simulink model "Mtest6"  (R2021b)
settings: Solver=FixedStepDiscrete  StartTime=0.0  StopTime=t_sim  FixedStep=0.01  RelTol=1e-3  EnableMultiTasking=on
model workspace (MAT data in the model file):
  SL_ROS_VariableLengthArrays_MaxSizes.CommonInfo.ArrayTruncateAction = 'EmitWarning'
  SL_ROS_VariableLengthArrays_MaxSizes.MsgTypeMap = containers.Map
  SL_ROS_VariableLengthArrays_MaxSizes.MsgTypeMap.serialization.keys = {'sensor_msgs/LaserScan'}
  SL_ROS_VariableLengthArrays_MaxSizes.MsgTypeMap.serialization.values{1}(1).PropertyName = 'Intensities'
  SL_ROS_VariableLengthArrays_MaxSizes.MsgTypeMap.serialization.values{1}(1).DataType = 'single'
  SL_ROS_VariableLengthArrays_MaxSizes.MsgTypeMap.serialization.values{1}(1).MaxLength = 360
  SL_ROS_VariableLengthArrays_MaxSizes.MsgTypeMap.serialization.values{1}(2).PropertyName = 'Ranges'
  SL_ROS_VariableLengthArrays_MaxSizes.MsgTypeMap.serialization.values{1}(2).DataType = 'single'
  SL_ROS_VariableLengthArrays_MaxSizes.MsgTypeMap.serialization.values{1}(2).MaxLength = 360
  SL_ROS_VariableLengthArrays_MaxSizes.MsgTypeMap.serialization.uniformity = 0
  SL_ROS_VariableLengthArrays_MaxSizes.MsgTypeMap.serialization.keyType = 'char'
  SL_ROS_VariableLengthArrays_MaxSizes.MsgTypeMap.serialization.valueType = 'any'
  rampa = 1
values from neighbouring files (symbols this model uses):
  x = x-0.1    [movimiento.m]
  y = y-0.1    [movimiento.m]
undefined symbols (not defined in the file or in its folder): a, Angular, Linear, rx1, rx2, rx3, ry1, ry2, ry3
libraries: robotlib x14, robotcorelib x3, robotalgslib x3, instrumentlib x1
settings Model: PacingRate=0.450000  Creator=The MathWorks, Inc.  LastModifiedBy=Cinthy
settings SolverCC: ConcurrentTasks=on  AlgebraicLoopSolver=TrustRegion  AutoInsertRateTranBlk=on
settings DataIOCC: LimitDataPoints=on  SaveFormat=StructureWithTime  ReturnWorkspaceOutputs=off
settings OptimizationCC: BlockReduction=off  EnhancedBackFolding=on  PassReuseOutputArgsAs=Individual arguments  ZeroExternalMemoryAtStartup=off  ZeroInternalMemoryAtStartup=off  MaxStackSize=64  OptimizeBlockOrder=speed  DifferentSizesBufferReuse=on  OptimizationCustomize=off  EfficientTunableParamExpr=on
settings DebuggingCC: SolverPrmCheckMsg=warning  ParameterTunabilityLossMsg=error  SFUnexpectedBacktrackingDiag=warning  SFNoUnconditionalDefaultTransitionDiag=warning  SFExecutionAtInitializationDiag=none  SFMachineParentedDataDiag=warning  ArithmeticOperatorsInVariantConditions=warning
settings HardwareCC: ProdBitPerPointer=32  ProdBitPerSizeT=32  ProdBitPerPtrDiffT=32  ProdLargestAtomicFloat=None  ProdIntDivRoundTo=Undefined  ProdEndianess=Unspecified  ProdWordSize=32  ProdHWDeviceType=Generic->Unspecified (assume 32-bit Generic)  TargetHWDeviceType=Generic->Unspecified (assume 32-bit Generic)
settings ModelReferenceCC: ModelReferenceNumInstancesAllowed=Single  PropagateSignalLabelsOutOfModel=off
settings SFSimCC: SimUseLocalCustomCode=off  MATLABDynamicMemAlloc=off  CustomCodeUndefinedFunction=UseInterfaceOnly  SimTargetLang=C++
settings RTWCC: Description=Embedded Coder  SystemTargetFile=ert.tlc  HardwareBoard=Robot Operating System (ROS)  TLCOptions="-aInlineSetEventsForThisBaseRateFcn=TLC_FALSE -aSuppressMultiTaskScheduler=TLC_FALSE  -aRateBasedStepFcn=0"  TemplateMakefile=ert_default_tmf  RTWUseLocalCustomCode=off  Toolchain=Catkin  TargetLang=C++
settings CodeAppCC: ForceParamTrailComments=on  IgnoreCustomStorageClasses=off  OperatorAnnotations=on  SimulinkDataObjDesc=on  SFDataObjDesc=on  InsertBlockDesc=on
settings ConfigComp: CovMetricSettings=dw  CovSaveCumulativeToWorkspaceVar=on  CovSaveSingleToWorkspaceVar=on  CovExternalEMLEnable=off  CovSFcnEnable=off

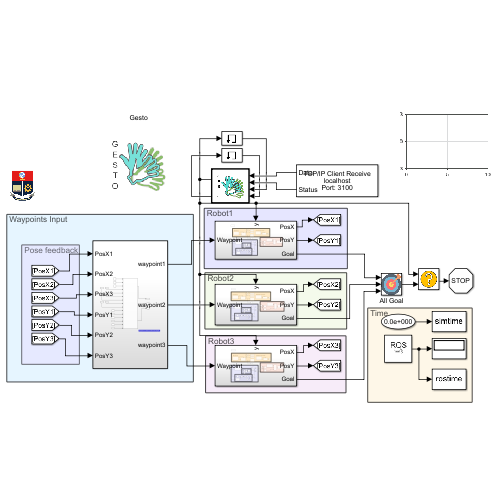
[thumbnail: Simulink's stored preview of the top-level diagram]
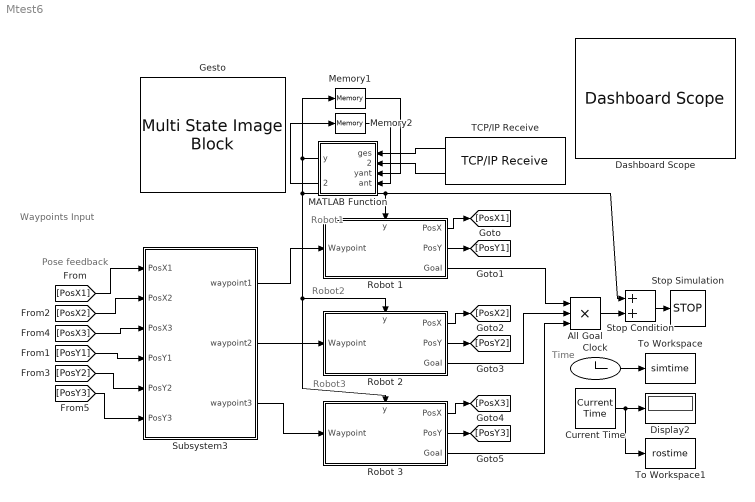
== system Mtest6 ==
  note: Time
  note: Pose feedback
  note: Robot3
  note: Robot2
  note: Robot1
  note: Waypoints Input
  All Goal : Product  Inputs=3  OutDataTypeStr=double
      mask Display: image('$imagefile'); % Use "Edit Image" on toolstrip to change.
  Clock : Clock
  Current Time : robotlib/Current Time  OutputFormat=double  SampleTime=-1  ModelName=Mtest6
      settings: SourceProductBaseCode=RR
  Dashboard Scope : DashboardScope  NormalizeYAxis=on
  Display2 : Display
  Gesto : MultiStateImageBlock  LabelPosition=Hide
  MATLAB Function : MATLAB Function  TreatAsAtomicUnit=on
  Memory1 : Memory
  Memory2 : Memory
  Robot 1 : Subsystem
      settings: PortSchema="{\"entries\":[{\"content\":{\"sides\":[{\"content\":{\"connectorIds\":[\"In1\"]},\"type\":\"ConnectorPlacement.EquallySpacedRectSide\",\"uuid\":\"ae525184-150a-424a-8495-0e96f94f0405\"},{\"content\":{\"connectorIds\":[\"Out1\",\"Out2\",\"Out3\"],\"side\":\"RIGHT\"},\"type\":\"ConnectorPlacement.EquallySpacedRectSide\",\"uuid\":\"56be0739-f54c-4565-abf9-53a283bf784a\"},{\"content\":{\"connectorIds\":[\"In2\"],\"side\":\"TOP\"},\"type\":\"ConnectorPlacement.EquallySpacedRectSide\",\"uuid\":\"def6bcfa-390a-4ec0-9486-bcadb35013bb\"}]},\"type\":\"ConnectorPlacement.EquallySpacedConnector\",\"uuid\":\"b414c082-bc88-4d09-823a-fc3316a4064c\"}],\"packageUris\":[\"http://schema.mathworks.com/mf0/Connector/R2020b\"],\"version\":\"1.0\"}"
  Robot 2 : Subsystem
      settings: PortSchema="{\"entries\":[{\"content\":{\"sides\":[{\"content\":{\"connectorIds\":[\"In1\"]},\"type\":\"ConnectorPlacement.EquallySpacedRectSide\",\"uuid\":\"ae525184-150a-424a-8495-0e96f94f0405\"},{\"content\":{\"connectorIds\":[\"Out1\",\"Out2\",\"Out3\"],\"side\":\"RIGHT\"},\"type\":\"ConnectorPlacement.EquallySpacedRectSide\",\"uuid\":\"56be0739-f54c-4565-abf9-53a283bf784a\"},{\"content\":{\"connectorIds\":[\"In2\"],\"side\":\"TOP\"},\"type\":\"ConnectorPlacement.EquallySpacedRectSide\",\"uuid\":\"def6bcfa-390a-4ec0-9486-bcadb35013bb\"}]},\"type\":\"ConnectorPlacement.EquallySpacedConnector\",\"uuid\":\"b414c082-bc88-4d09-823a-fc3316a4064c\"}],\"packageUris\":[\"http://schema.mathworks.com/mf0/Connector/R2020b\"],\"version\":\"1.0\"}"
  Robot 3 : Subsystem
      settings: PortSchema="{\"entries\":[{\"content\":{\"sides\":[{\"content\":{\"connectorIds\":[\"In1\"]},\"type\":\"ConnectorPlacement.EquallySpacedRectSide\",\"uuid\":\"ae525184-150a-424a-8495-0e96f94f0405\"},{\"content\":{\"connectorIds\":[\"Out1\",\"Out2\",\"Out3\"],\"side\":\"RIGHT\"},\"type\":\"ConnectorPlacement.EquallySpacedRectSide\",\"uuid\":\"56be0739-f54c-4565-abf9-53a283bf784a\"},{\"content\":{\"connectorIds\":[\"In2\"],\"side\":\"TOP\"},\"type\":\"ConnectorPlacement.EquallySpacedRectSide\",\"uuid\":\"def6bcfa-390a-4ec0-9486-bcadb35013bb\"}]},\"type\":\"ConnectorPlacement.EquallySpacedConnector\",\"uuid\":\"b414c082-bc88-4d09-823a-fc3316a4064c\"}],\"packageUris\":[\"http://schema.mathworks.com/mf0/Connector/R2020b\"],\"version\":\"1.0\"}"
  Stop Condition : Sum
      mask Display: image('$imagefile'); % Use "Edit Image" on toolstrip to change.
  Stop Simulation : Stop
  Subsystem3 : Subsystem
  TCP/IP Receive : instrumentlib/TCP//IP Receive  Host=localhost  Port=3100  DataSize=[ 1, 1 ]  DataType=uint8  ASCIIFormatting=%f  Terminator=LF  CustomTerminator=10  ByteOrder=big-endian  EnableBlockingMode=off  Timeout=10  SampleTime=0.1  SimulateUsing=Interpreted execution
  To Workspace : ToWorkspace  VariableName=simtime  SampleTime=-1
  To Workspace1 : ToWorkspace  VariableName=rostime  SampleTime=-1
  wires:
  Robot 1/1(PosX) -> [PosX1]
  Robot 1/2(PosY) -> [PosY1]
  Robot 2/1(PosX) -> [PosX2]
  Robot 2/2(PosY) -> [PosY2]
  Robot 3/1(PosX) -> [PosX3]
  Robot 3/2(PosY) -> [PosY3]
  Subsystem3/1(waypoint1) -> Robot 1/1(Waypoint)
  Subsystem3/2(waypoint2) -> Robot 2/1(Waypoint)
  Subsystem3/3(waypoint3) -> Robot 3/1(Waypoint)
  Robot 1/3(Goal) -> All Goal/1
  Robot 2/3(Goal) -> All Goal/2
  Robot 3/3(Goal) -> All Goal/3
  Clock/1 -> To Workspace/1
  [PosX1] -> Subsystem3/1(PosX1)
  [PosX2] -> Subsystem3/2(PosX2)
  [PosX3] -> Subsystem3/3(PosX3)
  [PosY1] -> Subsystem3/4(PosY1)
  [PosY2] -> Subsystem3/5(PosY2)
  [PosY3] -> Subsystem3/6(PosY3)
  Current Time/1 -> To Workspace1/1, Display2/1
  TCP/IP Receive/1 -> MATLAB Function/1(ges)
  MATLAB Function/1(y) -> Memory1/1, Robot 1/2(y), Stop Condition/1, Robot 2/2(y), Robot 3/2(y)
  All Goal/1 -> Stop Condition/2
  Stop Condition/1 -> Stop Simulation/1
  TCP/IP Receive/2 -> MATLAB Function/2(newData)
  MATLAB Function/2(gesto) -> Memory2/1
  Memory1/1 -> MATLAB Function/3(yant)
  Memory2/1 -> MATLAB Function/4(ant)

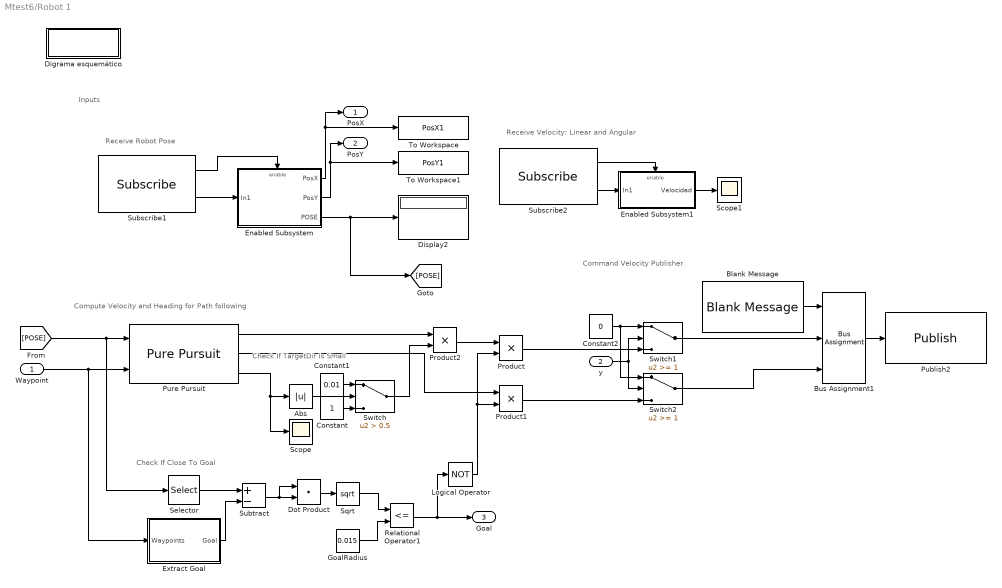
== system Mtest6/Robot 1 ==
  note: Check If TargetDir Is Small
  note: Compute Velocity and Heading for Path following
  note: Inputs
  note: Receive Robot Pose
  note: Check If Close To Goal
  note: Command Velocity Publisher
  note: Receive Velocity: Linear and Angular
  Waypoint : Inport
  y : Inport  Port=2
  " Extract Goal" : MATLAB Function  TreatAsAtomicUnit=on
  Abs : Abs
  Blank Message : robotlib/Blank Message  messageClass=Message  entityType=geometry_msgs/Twist  messageType=geometry_msgs/Twist  SampleTime=inf  legacyBusStruct=off
  Bus Assignment1 : BusAssignment  DialogController=Simulink.DDGSource_BusAssignment  AssignedSignals=Linear.X,Angular.Z
  Constant : Constant
  Constant1 : Constant  Value=0.01
  Constant2 : Constant  Value=0
  Digrama esquemático : Subsystem
  Display2 : Display
  Dot Product : DotProduct  InputSameDT=on  OutDataTypeStr=Inherit: Inherit via internal rule
  Enabled Subsystem : Subsystem
  Enabled Subsystem1 : Subsystem
  GoalRadius : Constant  Value=0.015
  Logical Operator : Logic  Operator=NOT  AllPortsSameDT=off  OutDataTypeStr=boolean
  Product : Product
  Product1 : Product
  Product2 : Product
  Publish2 : robotlib/Publish  topicSource=Select from ROS network  topic=/robot1/cmd_vel  messageType=geometry_msgs/Twist  legacyBusStruct=off  messageQueueLength=105
  Pure Pursuit : robotalgslib/Pure Pursuit  DesiredLinearVelocity=0.22  MaxAngularVelocity=2.84  LookaheadDistance=1.0  TargetDirPort=on  SimulateUsing=Code generation
  Relational Operator1 : RelationalOperator  Operator=<=  OutDataTypeStr=boolean  RndMeth=Simplest
  Scope : Scope
  Scope1 : Scope
  Selector : Selector  InputPortWidth=3  IndexOptions=Index vector (dialog)  Indices=[1 2]  OutputSizes=1
  Sqrt : Sqrt  SaturateOnIntegerOverflow=on
  Subscribe1 : robotlib/Subscribe  topicSource=Select from ROS network  topic=/robot1/odom  messageType=nav_msgs/Odometry  SampleTime=-1  legacyBusStruct=off  messageQueueLength=51
  Subscribe2 : robotlib/Subscribe  topicSource=Select from ROS network  topic=/robot1/cmd_vel  messageType=geometry_msgs/Twist  SampleTime=-1  legacyBusStruct=off  messageQueueLength=51
  Subtract : Sum  Inputs=+-
  Switch : Switch  Criteria=u2 > Threshold  Threshold=0.5
  Switch1 : Switch  Threshold=1
  Switch2 : Switch  Threshold=1
  To Workspace : ToWorkspace  VariableName=PosX1  SampleTime=-1
  To Workspace1 : ToWorkspace  VariableName=PosY1  SampleTime=-1
  PosX : Outport
  PosY : Outport  Port=2
  Goal : Outport  Port=3
  wires:
  GoalRadius/1 -> Relational Operator1/2
  Blank Message/1 -> Bus Assignment1/1
  Enabled Subsystem/3(POSE) -> [POSE], Display2/1
  Subtract/1 -> Dot Product/1, Dot Product/2
  Enabled Subsystem/2(PosY) -> PosY/1, To Workspace1/1
  Subscribe1/2 -> Enabled Subsystem/1(In1)
  Pure Pursuit/2 -> Product1/1
  Subscribe1/1 -> Enabled Subsystem/Enable
  Enabled Subsystem/1(PosX) -> PosX/1, To Workspace/1
  Relational Operator1/1 -> Logical Operator/1, Goal/1
  Bus Assignment1/1 -> Publish2/1
  [POSE] -> Selector/1, Pure Pursuit/1
  Dot Product/1 -> Sqrt/1
  " Extract Goal"/1(Goal) -> Subtract/2
  Selector/1 -> Subtract/1
  Sqrt/1 -> Relational Operator1/1
  Logical Operator/1 -> Product/2, Product1/2
  Waypoint/1 -> " Extract Goal"/1(Waypoints), Pure Pursuit/2
  Pure Pursuit/3 -> Scope/1, Abs/1
  Constant/1 -> Switch/3
  Constant1/1 -> Switch/1
  Switch/1 -> Product2/2
  Product2/1 -> Product/1
  Abs/1 -> Switch/2
  Pure Pursuit/1 -> Product2/1
  y/1 -> Switch1/2, Switch2/2
  Constant2/1 -> Switch2/1, Switch1/1
  Product/1 -> Switch1/3
  Product1/1 -> Switch2/3
  Switch1/1 -> Bus Assignment1/2
  Switch2/1 -> Bus Assignment1/3
  Subscribe2/2 -> Enabled Subsystem1/1(In1)
  Subscribe2/1 -> Enabled Subsystem1/Enable
  Enabled Subsystem1/1(Velocidad) -> Scope1/1

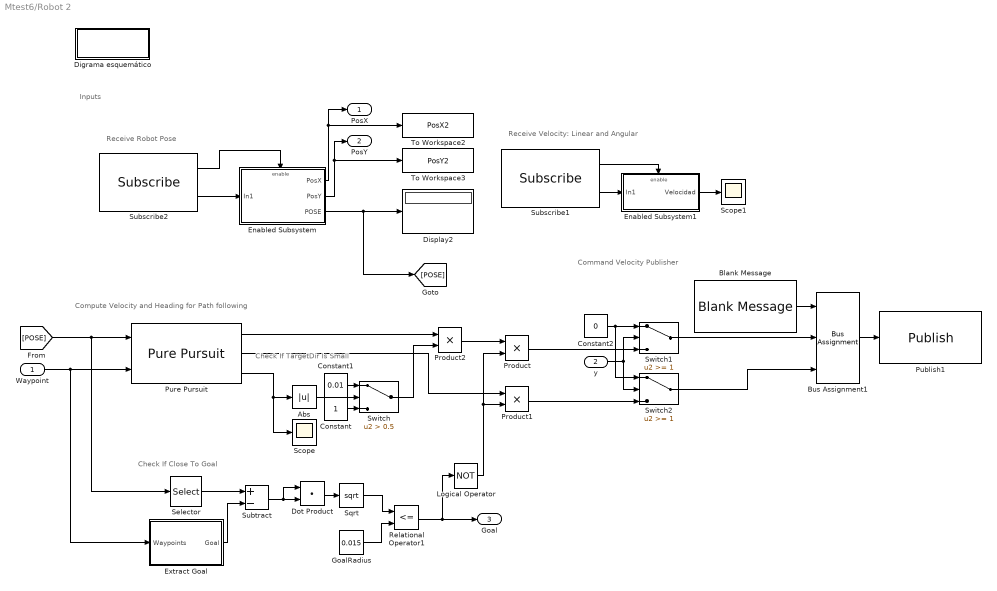
== system Mtest6/Robot 2 ==
  note: Check If TargetDir Is Small
  note: Compute Velocity and Heading for Path following
  note: Inputs
  note: Receive Robot Pose
  note: Check If Close To Goal
  note: Command Velocity Publisher
  note: Receive Velocity: Linear and Angular
  Waypoint : Inport
  y : Inport  Port=2
  " Extract Goal" : MATLAB Function  TreatAsAtomicUnit=on
  Abs : Abs
  Blank Message : robotlib/Blank Message  messageClass=Message  entityType=geometry_msgs/Twist  messageType=geometry_msgs/Twist  SampleTime=inf  legacyBusStruct=off
  Bus Assignment1 : BusAssignment  DialogController=Simulink.DDGSource_BusAssignment  AssignedSignals=Linear.X,Angular.Z
  Constant : Constant
  Constant1 : Constant  Value=0.01
  Constant2 : Constant  Value=0
  Digrama esquemático : Subsystem
  Display2 : Display
  Dot Product : DotProduct  InputSameDT=on  OutDataTypeStr=Inherit: Inherit via internal rule
  Enabled Subsystem : Subsystem
  Enabled Subsystem1 : Subsystem
  GoalRadius : Constant  Value=0.015
  Logical Operator : Logic  Operator=NOT  AllPortsSameDT=off  OutDataTypeStr=boolean
  Product : Product
  Product1 : Product
  Product2 : Product
  Publish1 : robotlib/Publish  topicSource=Select from ROS network  topic=/robot2/cmd_vel  messageType=geometry_msgs/Twist  legacyBusStruct=off  messageQueueLength=105
  Pure Pursuit : robotalgslib/Pure Pursuit  DesiredLinearVelocity=0.22  MaxAngularVelocity=2.84  LookaheadDistance=1.0  TargetDirPort=on  SimulateUsing=Code generation
  Relational Operator1 : RelationalOperator  Operator=<=  OutDataTypeStr=boolean  RndMeth=Simplest
  Scope : Scope
  Scope1 : Scope
  Selector : Selector  InputPortWidth=3  IndexOptions=Index vector (dialog)  Indices=[1 2]  OutputSizes=1
  Sqrt : Sqrt  SaturateOnIntegerOverflow=on
  Subscribe1 : robotlib/Subscribe  topicSource=Select from ROS network  topic=/robot2/cmd_vel  messageType=geometry_msgs/Twist  SampleTime=-1  legacyBusStruct=off  messageQueueLength=51
  Subscribe2 : robotlib/Subscribe  topicSource=Select from ROS network  topic=/robot2/odom  messageType=nav_msgs/Odometry  SampleTime=-1  legacyBusStruct=off  messageQueueLength=51
  Subtract : Sum  Inputs=+-
  Switch : Switch  Criteria=u2 > Threshold  Threshold=0.5
  Switch1 : Switch  Threshold=1
  Switch2 : Switch  Threshold=1
  To Workspace2 : ToWorkspace  VariableName=PosX2  SampleTime=-1
  To Workspace3 : ToWorkspace  VariableName=PosY2  SampleTime=-1
  PosX : Outport
  PosY : Outport  Port=2
  Goal : Outport  Port=3
  wires:
  GoalRadius/1 -> Relational Operator1/2
  Blank Message/1 -> Bus Assignment1/1
  Enabled Subsystem/3(POSE) -> [POSE], Display2/1
  Subtract/1 -> Dot Product/1, Dot Product/2
  Enabled Subsystem/2(PosY) -> To Workspace3/1, PosY/1
  Subscribe2/2 -> Enabled Subsystem/1(In1)
  Pure Pursuit/2 -> Product1/1
  Subscribe2/1 -> Enabled Subsystem/Enable
  Enabled Subsystem/1(PosX) -> To Workspace2/1, PosX/1
  Relational Operator1/1 -> Logical Operator/1, Goal/1
  Bus Assignment1/1 -> Publish1/1
  [POSE] -> Selector/1, Pure Pursuit/1
  Dot Product/1 -> Sqrt/1
  " Extract Goal"/1(Goal) -> Subtract/2
  Selector/1 -> Subtract/1
  Sqrt/1 -> Relational Operator1/1
  Logical Operator/1 -> Product/2, Product1/2
  Waypoint/1 -> " Extract Goal"/1(Waypoints), Pure Pursuit/2
  Pure Pursuit/3 -> Scope/1, Abs/1
  Constant/1 -> Switch/3
  Constant1/1 -> Switch/1
  Switch/1 -> Product2/2
  Product2/1 -> Product/1
  Abs/1 -> Switch/2
  Pure Pursuit/1 -> Product2/1
  Product1/1 -> Switch2/3
  y/1 -> Switch1/2, Switch2/2
  Constant2/1 -> Switch2/1, Switch1/1
  Product/1 -> Switch1/3
  Switch1/1 -> Bus Assignment1/2
  Switch2/1 -> Bus Assignment1/3
  Subscribe1/1 -> Enabled Subsystem1/Enable
  Subscribe1/2 -> Enabled Subsystem1/1(In1)
  Enabled Subsystem1/1(Velocidad) -> Scope1/1

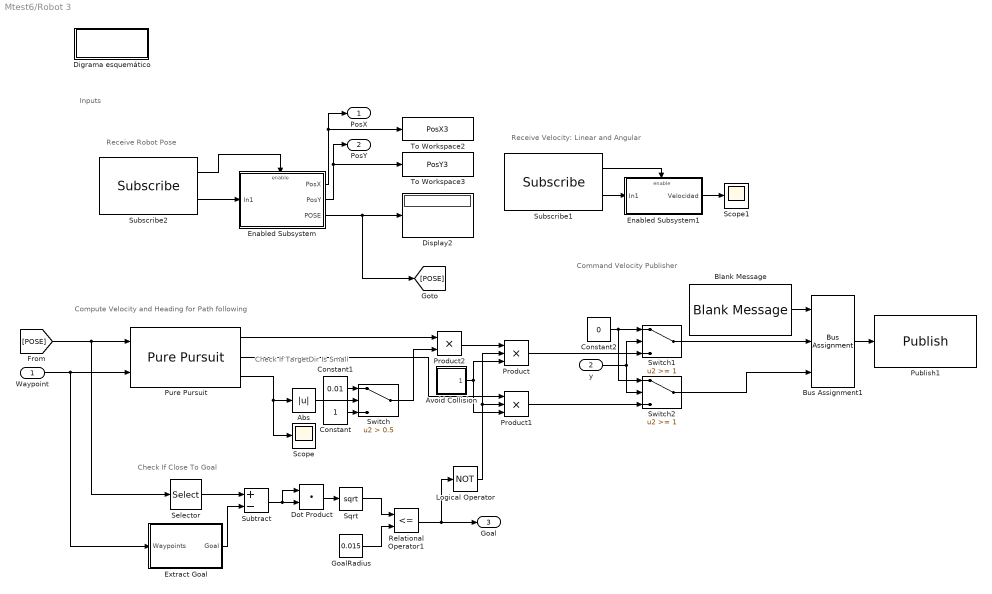
== system Mtest6/Robot 3 ==
  note: Check If TargetDir Is Small
  note: Compute Velocity and Heading for Path following
  note: Inputs
  note: Receive Robot Pose
  note: Check If Close To Goal
  note: Command Velocity Publisher
  note: Receive Velocity: Linear and Angular
  Waypoint : Inport
  y : Inport  Port=2
  " Extract Goal" : MATLAB Function  TreatAsAtomicUnit=on
  Abs : Abs
  Avoid Collision : Subsystem
  Blank Message : robotlib/Blank Message  messageClass=Message  entityType=geometry_msgs/Twist  messageType=geometry_msgs/Twist  SampleTime=inf  legacyBusStruct=off
  Bus Assignment1 : BusAssignment  DialogController=Simulink.DDGSource_BusAssignment  AssignedSignals=Linear.X,Angular.Z
  Constant : Constant
  Constant1 : Constant  Value=0.01
  Constant2 : Constant  Value=0
  Digrama esquemático : Subsystem
  Display2 : Display
  Dot Product : DotProduct  InputSameDT=on  OutDataTypeStr=Inherit: Inherit via internal rule
  Enabled Subsystem : Subsystem
  Enabled Subsystem1 : Subsystem
  GoalRadius : Constant  Value=0.015
  Logical Operator : Logic  Operator=NOT  AllPortsSameDT=off  OutDataTypeStr=boolean
  Product : Product  Inputs=3
  Product1 : Product  Inputs=3
  Product2 : Product
  Publish1 : robotlib/Publish  topicSource=Select from ROS network  topic=/robot3/cmd_vel  messageType=geometry_msgs/Twist  legacyBusStruct=off  messageQueueLength=105
  Pure Pursuit : robotalgslib/Pure Pursuit  DesiredLinearVelocity=0.22  MaxAngularVelocity=2.84  LookaheadDistance=1.0  TargetDirPort=on  SimulateUsing=Code generation
  Relational Operator1 : RelationalOperator  Operator=<=  OutDataTypeStr=boolean  RndMeth=Simplest
  Scope : Scope
  Scope1 : Scope
  Selector : Selector  InputPortWidth=3  IndexOptions=Index vector (dialog)  Indices=[1 2]  OutputSizes=1
  Sqrt : Sqrt  SaturateOnIntegerOverflow=on
  Subscribe1 : robotlib/Subscribe  topicSource=Select from ROS network  topic=/robot3/cmd_vel  messageType=geometry_msgs/Twist  SampleTime=-1  legacyBusStruct=off  messageQueueLength=51
  Subscribe2 : robotlib/Subscribe  topicSource=Select from ROS network  topic=/robot3/odom  messageType=nav_msgs/Odometry  SampleTime=-1  legacyBusStruct=off  messageQueueLength=51
  Subtract : Sum  Inputs=+-
  Switch : Switch  Criteria=u2 > Threshold  Threshold=0.5
  Switch1 : Switch  Threshold=1
  Switch2 : Switch  Threshold=1
  To Workspace2 : ToWorkspace  VariableName=PosX3  SampleTime=-1
  To Workspace3 : ToWorkspace  VariableName=PosY3  SampleTime=-1
  PosX : Outport
  PosY : Outport  Port=2
  Goal : Outport  Port=3
  wires:
  GoalRadius/1 -> Relational Operator1/2
  Blank Message/1 -> Bus Assignment1/1
  Enabled Subsystem/3(POSE) -> [POSE], Display2/1
  Subtract/1 -> Dot Product/1, Dot Product/2
  Enabled Subsystem/2(PosY) -> To Workspace3/1, PosY/1
  Subscribe2/2 -> Enabled Subsystem/1(In1)
  Pure Pursuit/2 -> Product1/1
  Subscribe2/1 -> Enabled Subsystem/Enable
  Enabled Subsystem/1(PosX) -> To Workspace2/1, PosX/1
  Relational Operator1/1 -> Logical Operator/1, Goal/1
  Bus Assignment1/1 -> Publish1/1
  [POSE] -> Selector/1, Pure Pursuit/1
  Dot Product/1 -> Sqrt/1
  " Extract Goal"/1(Goal) -> Subtract/2
  Selector/1 -> Subtract/1
  Sqrt/1 -> Relational Operator1/1
  Logical Operator/1 -> Product/2, Product1/2
  Waypoint/1 -> " Extract Goal"/1(Waypoints), Pure Pursuit/2
  Pure Pursuit/3 -> Scope/1, Abs/1
  Constant/1 -> Switch/3
  Constant1/1 -> Switch/1
  Switch/1 -> Product2/2
  Product2/1 -> Product/1
  Abs/1 -> Switch/2
  Pure Pursuit/1 -> Product2/1
  Product/1 -> Switch1/3
  Product1/1 -> Switch2/3
  Constant2/1 -> Switch2/1, Switch1/1
  y/1 -> Switch1/2, Switch2/2
  Switch1/1 -> Bus Assignment1/2
  Switch2/1 -> Bus Assignment1/3
  Subscribe1/1 -> Enabled Subsystem1/Enable
  Subscribe1/2 -> Enabled Subsystem1/1(In1)
  Enabled Subsystem1/1(Velocidad) -> Scope1/1
  Avoid Collision/1(noStop) -> Product1/3, Product/3

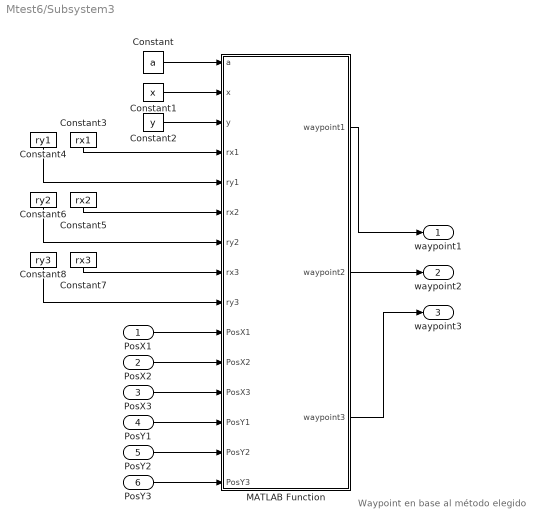
== system Mtest6/Subsystem3 ==
  note: Waypoint en base al método elegido
  PosX1 : Inport
  PosX2 : Inport  Port=2
  PosX3 : Inport  Port=3
  PosY1 : Inport  Port=4
  PosY2 : Inport  Port=5
  PosY3 : Inport  Port=6
  Constant : Constant  Value=a
  Constant1 : Constant  Value=x
  Constant2 : Constant  Value=y
  Constant3 : Constant  Value=rx1
  Constant4 : Constant  Value=ry1
  Constant5 : Constant  Value=rx2
  Constant6 : Constant  Value=ry2
  Constant7 : Constant  Value=rx3
  Constant8 : Constant  Value=ry3
  MATLAB Function : MATLAB Function  TreatAsAtomicUnit=on
  waypoint1 : Outport
  waypoint2 : Outport  Port=2
  waypoint3 : Outport  Port=3
  wires:
  PosY3/1 -> MATLAB Function/15(PosY3)
  MATLAB Function/2(waypoint2) -> waypoint2/1
  Constant/1 -> MATLAB Function/1(a)
  Constant2/1 -> MATLAB Function/3(y)
  Constant1/1 -> MATLAB Function/2(x)
  Constant7/1 -> MATLAB Function/8(rx3)
  MATLAB Function/3(waypoint3) -> waypoint3/1
  PosX1/1 -> MATLAB Function/10(PosX1)
  PosY2/1 -> MATLAB Function/14(PosY2)
  Constant6/1 -> MATLAB Function/7(ry2)
  PosX3/1 -> MATLAB Function/12(PosX3)
  PosX2/1 -> MATLAB Function/11(PosX2)
  MATLAB Function/1(waypoint1) -> waypoint1/1
  PosY1/1 -> MATLAB Function/13(PosY1)
  Constant8/1 -> MATLAB Function/9(ry3)
  Constant3/1 -> MATLAB Function/4(rx1)
  Constant4/1 -> MATLAB Function/5(ry1)
  Constant5/1 -> MATLAB Function/6(rx2)

== system Mtest6/Robot 1/Digrama esquemático ==
  note: Definición de Velocidad lineal y angular
  note: >
  note: _____
  note: Waypoint
  note: |
      | |
      | |
  note: / |
      | [POSE] |
      | \_______|
  note: ______|
  note: Definir mensaje a enviar
  note: Comprobar si llegó a la meta
  note: Condiconamiento de Velocidad lineal
  note: Envio Velocidades al Robot
  note: Control Pure Pursuit
  note: Visualización
  note: Procesamiento de datos
  note: Recibir Pose del Robot
  note: | \
      | | [POSE]
      | |_______/
  note: >
  note: _____
  note: >
  note: _____
  note: _____
  note: >
  note: _____
  note: >
  note: _____
  note: >
  note: >
  note: _____
  note: >
  note: _____
  note: __________________
  note: >
  note: _____
  note: >
  note: _____
  note: >
  note: |
  note: >
  note: ____________________
  note: |
  note: >
  note: ___
  note: |
  note: |
  note: |
  note: ___
  note: _______________________________
  note: >
  note: ___
  note: |
  note: >
  note: _____
  note: |
  note: |
  note: |
  note: |
  note: |
  note: |
  note: |
  note: |
  note: |
  note: |
  note: |
  note: |
  note: |
  note: |
  note: |
  note: |

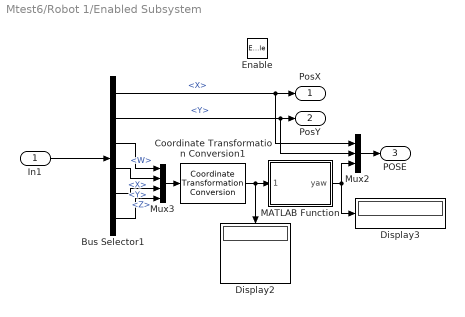
== system Mtest6/Robot 1/Enabled Subsystem ==
  In1 : Inport
  Enable : EnablePort
  Bus Selector1 : BusSelector  DialogController=Simulink.DDGSource_BusSelector  OutputSignals=Pose.Pose.Position.X,Pose.Pose.Position.Y,Pose.Pose.Orientation.W,Pose.Pose.Orientation.X,Pose.Pose.Orientation.Y,Pose.Pose.Orientation.Z
  Coordinate Transformation Conversion1 : robotcorelib/Coordinate Transformation Conversion  InputRepresentation=Quaternion  InputEulerSequence=ZYX  ShowTrVecInputPort=on  OutputRepresentation=Euler Angles  OutputEulerSequence=ZYX  ShowTrVecOutputPort=on  SimulateUsing=Interpreted execution
      settings: SourceProductBaseCode=NV,RO,RR,UV
  Display2 : Display
  Display3 : Display
  MATLAB Function : MATLAB Function  TreatAsAtomicUnit=on
  Mux2 : Mux  Inputs=3
  Mux3 : Mux
  PosX : Outport  VectorParamsAs1DForOutWhenUnconnected=off
  PosY : Outport  Port=2  VectorParamsAs1DForOutWhenUnconnected=off
  POSE : Outport  Port=3
  wires:
  MATLAB Function/1(yaw) -> Mux2/3, Display3/1
  Bus Selector1/6 -> Mux3/4  "<Z>"
  Mux3/1 -> Coordinate Transformation Conversion1/1
  Bus Selector1/2 -> Mux2/2, PosY/1  "<Y>"
  Bus Selector1/4 -> Mux3/2  "<X>"
  Coordinate Transformation Conversion1/1 -> Display2/1, MATLAB Function/1(eulerAng)
  Bus Selector1/3 -> Mux3/1  "<W>"
  Mux2/1 -> POSE/1
  In1/1 -> Bus Selector1/1
  Bus Selector1/5 -> Mux3/3  "<Y>"
  Bus Selector1/1 -> PosX/1, Mux2/1  "<X>"

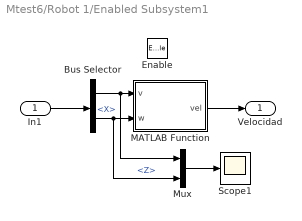
== system Mtest6/Robot 1/Enabled Subsystem1 ==
  In1 : Inport
  Enable : EnablePort
  Bus Selector : BusSelector  DialogController=Simulink.DDGSource_BusSelector  OutputSignals=Linear.X,Angular.Z
  MATLAB Function : MATLAB Function  TreatAsAtomicUnit=on
  Mux : Mux  Inputs=2
  Scope1 : Scope
  Velocidad : Outport  VectorParamsAs1DForOutWhenUnconnected=off
  wires:
  In1/1 -> Bus Selector/1
  Bus Selector/1 -> Mux/1, MATLAB Function/1(v)  "<X>"
  Bus Selector/2 -> Mux/2, MATLAB Function/2(w)  "<Z>"
  MATLAB Function/1(vel) -> Velocidad/1
  Mux/1 -> Scope1/1

== system Mtest6/Robot 2/Digrama esquemático ==
  note: Definición de Velocidad lineal y angular
  note: >
  note: _____
  note: Waypoint
  note: |
      | |
      | |
  note: / |
      | [POSE] |
      | \_______|
  note: ______|
  note: Definir mensaje a enviar
  note: Comprobar si llegó a la meta
  note: Condiconamiento de Velocidad lineal
  note: Envio Velocidades al Robot
  note: Control Pure Pursuit
  note: Visualización
  note: Procesamiento de datos
  note: Recibir Pose del Robot
  note: | \
      | | [POSE]
      | |_______/
  note: >
  note: _____
  note: >
  note: _____
  note: _____
  note: >
  note: _____
  note: >
  note: _____
  note: >
  note: >
  note: _____
  note: >
  note: _____
  note: __________________
  note: >
  note: _____
  note: >
  note: _____
  note: >
  note: |
  note: >
  note: ____________________
  note: |
  note: >
  note: ___
  note: |
  note: |
  note: |
  note: ___
  note: _______________________________
  note: >
  note: ___
  note: |
  note: >
  note: _____
  note: |
  note: |
  note: |
  note: |
  note: |
  note: |
  note: |
  note: |
  note: |
  note: |
  note: |
  note: |
  note: |
  note: |
  note: |
  note: |

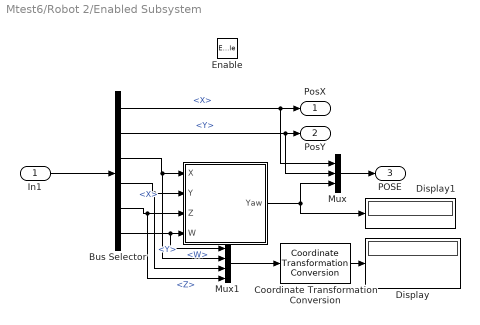
== system Mtest6/Robot 2/Enabled Subsystem ==
  In1 : Inport
  Enable : EnablePort
  " " : MATLAB Function  TreatAsAtomicUnit=on
  Bus Selector : BusSelector  DialogController=Simulink.DDGSource_BusSelector  OutputSignals=Pose.Pose.Position.X,Pose.Pose.Position.Y,Pose.Pose.Orientation.X,Pose.Pose.Orientation.Y,Pose.Pose.Orientation.Z,Pose.Pose.Orientation.W
  Coordinate Transformation Conversion : robotcorelib/Coordinate Transformation Conversion  InputRepresentation=Quaternion  InputEulerSequence=ZYX  ShowTrVecInputPort=on  OutputRepresentation=Euler Angles  OutputEulerSequence=XYZ  ShowTrVecOutputPort=on  SimulateUsing=Interpreted execution
      settings: SourceProductBaseCode=NV,RO,RR,UV
  Display : Display
  Display1 : Display
  Mux : Mux  Inputs=3
  Mux1 : Mux
  PosX : Outport  VectorParamsAs1DForOutWhenUnconnected=off
  PosY : Outport  Port=2  VectorParamsAs1DForOutWhenUnconnected=off
  POSE : Outport  Port=3
  wires:
  In1/1 -> Bus Selector/1
  Bus Selector/2 -> Mux/2, PosY/1  "<Y>"
  Bus Selector/1 -> Mux/1, PosX/1  "<X>"
  Bus Selector/3 -> Mux1/2, " "/1(X)  "<X>"
  Bus Selector/4 -> Mux1/3, " "/2(Y)  "<Y>"
  Bus Selector/5 -> Mux1/4, " "/3(Z)  "<Z>"
  Bus Selector/6 -> Mux1/1, " "/4(W)  "<W>"
  " "/1(Yaw) -> Mux/3, Display1/1
  Mux/1 -> POSE/1
  Coordinate Transformation Conversion/1 -> Display/1
  Mux1/1 -> Coordinate Transformation Conversion/1

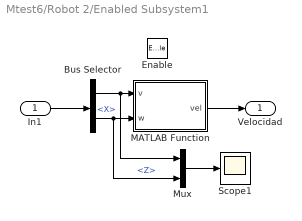
== system Mtest6/Robot 2/Enabled Subsystem1 ==
  In1 : Inport
  Enable : EnablePort
  Bus Selector : BusSelector  DialogController=Simulink.DDGSource_BusSelector  OutputSignals=Linear.X,Angular.Z
  MATLAB Function : MATLAB Function  TreatAsAtomicUnit=on
  Mux : Mux  Inputs=2
  Scope1 : Scope
  Velocidad : Outport  VectorParamsAs1DForOutWhenUnconnected=off
  wires:
  In1/1 -> Bus Selector/1
  Bus Selector/1 -> Mux/1, MATLAB Function/1(v)  "<X>"
  Bus Selector/2 -> Mux/2, MATLAB Function/2(w)  "<Z>"
  MATLAB Function/1(vel) -> Velocidad/1
  Mux/1 -> Scope1/1

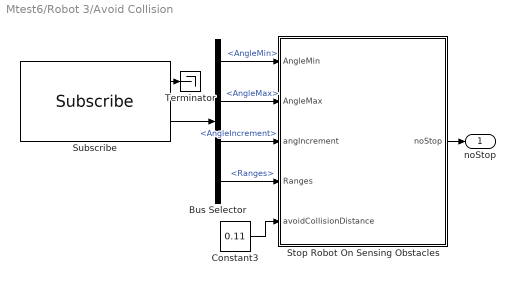
== system Mtest6/Robot 3/Avoid Collision ==
  Bus Selector : BusSelector  OutputSignals=AngleMin,AngleMax,AngleIncrement,Ranges
  Constant3 : Constant  Value=0.11
  Stop Robot On Sensing Obstacles : MATLAB Function  TreatAsAtomicUnit=on
  Subscribe : robotlib/Subscribe  topicSource=Select from ROS network  topic=/robot3/scan  messageType=sensor_msgs/LaserScan  SampleTime=-1  legacyBusStruct=off  messageQueueLength=1
  Terminator : Terminator
  noStop : Outport
  wires:
  Constant3/1 -> Stop Robot On Sensing Obstacles/5(avoidCollisionDistance)
  Subscribe/2 -> Bus Selector/1
  Subscribe/1 -> Terminator/1
  Bus Selector/4 -> Stop Robot On Sensing Obstacles/4(Ranges)  "<Ranges>"
  Bus Selector/2 -> Stop Robot On Sensing Obstacles/2(AngleMax)  "<AngleMax>"
  Bus Selector/3 -> Stop Robot On Sensing Obstacles/3(angIncrement)  "<AngleIncrement>"
  Stop Robot On Sensing Obstacles/1(noStop) -> noStop/1
  Bus Selector/1 -> Stop Robot On Sensing Obstacles/1(AngleMin)  "<AngleMin>"

== system Mtest6/Robot 3/Digrama esquemático ==
  note: Definición de Velocidad lineal y angular
  note: >
  note: _____
  note: Waypoint
  note: |
      | |
      | |
  note: / |
      | [POSE] |
      | \_______|
  note: ______|
  note: Definir mensaje a enviar
  note: Comprobar si llegó a la meta
  note: Condiconamiento de Velocidad lineal
  note: Envio Velocidades al Robot
  note: Control Pure Pursuit
  note: Visualización
  note: Procesamiento de datos
  note: Recibir Pose del Robot
  note: | \
      | | [POSE]
      | |_______/
  note: >
  note: _____
  note: >
  note: _____
  note: _____
  note: >
  note: _____
  note: >
  note: _____
  note: >
  note: >
  note: _____
  note: >
  note: _____
  note: __________________
  note: >
  note: _____
  note: >
  note: _____
  note: >
  note: |
  note: >
  note: ____________________
  note: |
  note: >
  note: ___
  note: |
  note: |
  note: |
  note: ___
  note: _______________________________
  note: >
  note: ___
  note: |
  note: >
  note: _____
  note: |
  note: |
  note: |
  note: |
  note: |
  note: |
  note: |
  note: |
  note: |
  note: |
  note: |
  note: |
  note: |
  note: |
  note: |
  note: |

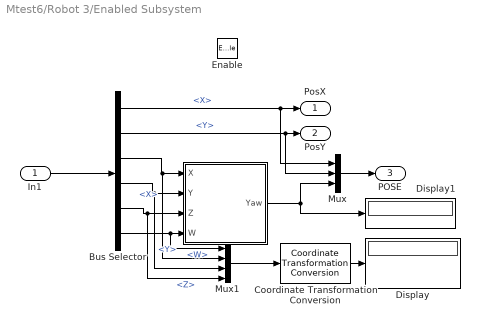
== system Mtest6/Robot 3/Enabled Subsystem ==
  In1 : Inport
  Enable : EnablePort
  " " : MATLAB Function  TreatAsAtomicUnit=on
  Bus Selector : BusSelector  DialogController=Simulink.DDGSource_BusSelector  OutputSignals=Pose.Pose.Position.X,Pose.Pose.Position.Y,Pose.Pose.Orientation.X,Pose.Pose.Orientation.Y,Pose.Pose.Orientation.Z,Pose.Pose.Orientation.W
  Coordinate Transformation Conversion : robotcorelib/Coordinate Transformation Conversion  InputRepresentation=Quaternion  InputEulerSequence=ZYX  ShowTrVecInputPort=on  OutputRepresentation=Euler Angles  OutputEulerSequence=XYZ  ShowTrVecOutputPort=on  SimulateUsing=Interpreted execution
      settings: SourceProductBaseCode=NV,RO,RR,UV
  Display : Display
  Display1 : Display
  Mux : Mux  Inputs=3
  Mux1 : Mux
  PosX : Outport  VectorParamsAs1DForOutWhenUnconnected=off
  PosY : Outport  Port=2  VectorParamsAs1DForOutWhenUnconnected=off
  POSE : Outport  Port=3
  wires:
  In1/1 -> Bus Selector/1
  Bus Selector/2 -> Mux/2, PosY/1  "<Y>"
  Bus Selector/1 -> Mux/1, PosX/1  "<X>"
  Bus Selector/3 -> Mux1/2, " "/1(X)  "<X>"
  Bus Selector/4 -> Mux1/3, " "/2(Y)  "<Y>"
  Bus Selector/5 -> Mux1/4, " "/3(Z)  "<Z>"
  Bus Selector/6 -> Mux1/1, " "/4(W)  "<W>"
  " "/1(Yaw) -> Mux/3, Display1/1
  Mux/1 -> POSE/1
  Coordinate Transformation Conversion/1 -> Display/1
  Mux1/1 -> Coordinate Transformation Conversion/1

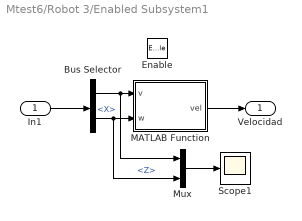
== system Mtest6/Robot 3/Enabled Subsystem1 ==
  In1 : Inport
  Enable : EnablePort
  Bus Selector : BusSelector  DialogController=Simulink.DDGSource_BusSelector  OutputSignals=Linear.X,Angular.Z
  MATLAB Function : MATLAB Function  TreatAsAtomicUnit=on
  Mux : Mux  Inputs=2
  Scope1 : Scope
  Velocidad : Outport  VectorParamsAs1DForOutWhenUnconnected=off
  wires:
  In1/1 -> Bus Selector/1
  Bus Selector/1 -> Mux/1, MATLAB Function/1(v)  "<X>"
  Bus Selector/2 -> Mux/2, MATLAB Function/2(w)  "<Z>"
  MATLAB Function/1(vel) -> Velocidad/1
  Mux/1 -> Scope1/1

== matlab function Mtest6/Robot 2/ Extract Goal ==
  data: Waypoints input; Goal output
function Goal = extractGoal(Waypoints)
%#codegen
b = isnan(Waypoints);
[rows,~] = find(b);
ridx = setdiff(1:size(Waypoints,1), sort(rows));
Goal = [Waypoints(ridx(end), 1) Waypoints(ridx(end), 2)];

== matlab function Mtest6/Robot 2/Enabled Subsystem/  ==
  data: X input; Yaw output; Y input; Z input; W input
function Yaw = quat2eulBlk(X, Y, Z, W)
%#codegen

eularAngles = quat2eul([W, X, Y, Z]);
Yaw = eularAngles(1);

== matlab function Mtest6/Robot 3/ Extract Goal ==
  data: Waypoints input; Goal output
function Goal = extractGoal(Waypoints)
%#codegen
b = isnan(Waypoints);
[rows,~] = find(b);
ridx = setdiff(1:size(Waypoints,1), sort(rows));
Goal = [Waypoints(ridx(end), 1) Waypoints(ridx(end), 2)];

== matlab function Mtest6/Robot 3/Enabled Subsystem/  ==
  data: X input; Yaw output; Y input; Z input; W input
function Yaw = quat2eulBlk(X, Y, Z, W)
%#codegen

eularAngles = quat2eul([W, X, Y, Z]);
Yaw = eularAngles(1);

== matlab function Mtest6/Robot 1/Enabled Subsystem1/MATLAB Function ==
  data: v input; vel output; w input
function vel = fcn(v,w)

vel = sqrt(v^2+w^2);

== matlab function Mtest6/MATLAB Function ==
  data: ges input; y output; newData input; gesto output double; yant input; ant input
function [y,gesto]  = stop(ges,newData,yant,ant)
% coder.extrinsic('Simulink.Annotation')
if newData==1
    gesto=double(ges);
    if ges==4%open
        y=1;
    %     switch ges
    %         case 1
    %             gesto = 'Wave Out';
    %         case 2
    %             gesto = 'Wave In';
    %         case 3
    %             gesto = 'Fist';
    %         case 4
    %             gesto = 'Open';
    %         case 5
    %             gesto = 'Pinch';
    %         otherwise
    %             gesto = 'No gesture';
    %     end
    else
        y=0;
    end
    % a = Simulink.Annotation('Mtest6/GESTO');
    
    % setImage(Simulink.Annotation('Mtest6/GESTO'),img)
else
    gesto=ant;
    y=yant;
end

== matlab function Mtest6/Robot 1/Enabled Subsystem/MATLAB Function ==
  data: eulerAng input; yaw output
function yaw = fcn(eulerAng)

yaw = eulerAng(1);

== matlab function Mtest6/Robot 2/Enabled Subsystem1/MATLAB Function ==
  data: v input; vel output; w input
function vel = fcn(v,w)

vel = sqrt(v^2+w^2);

== matlab function Mtest6/Robot 3/Enabled Subsystem1/MATLAB Function ==
  data: v input; vel output; w input
function vel = fcn(v,w)

vel = sqrt(v^2+w^2);

== matlab function Mtest6/Subsystem3/MATLAB Function ==
  data: a input; x input; y input; rx1 input; ry1 input; rx2 input; ry2 input; rx3 input; ry3 input; waypoint1 output; waypoint2 output; waypoint3 output; PosX1 input; PosX2 input; PosX3 input; PosY1 input; PosY2 input; PosY3 input
function [waypoint1,waypoint2,waypoint3] = waypoint_metod(a,x,y,rx1,ry1,rx2,ry2,rx3,ry3,PosX1,PosX2,PosX3,PosY1,PosY2,PosY3)
%a=3 Metodo 1,a=4 Metodo 2, else Inicializacion,a=2 One_Robot

if a==3
    waypoint1=[PosX1(length(PosX1)) PosY1(length(PosY1));x+rx1 y+ry1];
    waypoint2=[PosX2(length(PosX2)) PosY2(length(PosY2));x+rx2 y+ry2];
    waypoint3=[PosX3(length(PosX3)) PosY3(length(PosY3));x+rx3 y+ry3];
elseif a==4
    waypoint1=[PosX1(length(PosX1)) PosY1(length(PosY1));PosX2(length(PosX2))+rx1-rx2 PosY2(length(PosY2))+ry1-ry2];
    waypoint2=[PosX2(length(PosX2)) PosY2(length(PosY2));x+rx2 y+ry2];
    waypoint3=[PosX3(length(PosX3)) PosY3(length(PosY3));PosX2(length(PosX2))+rx3-rx2 PosY2(length(PosY2))+ry3-ry2];  
elseif a==2
    waypoint1=[PosX1(length(PosX1)) PosY1(length(PosY1));x+rx1 y+ry1];
    waypoint2=[PosX2(length(PosX2)) PosY2(length(PosY2));PosX2(length(PosX2)) PosY2(length(PosY2))];
    waypoint3=[PosX3(length(PosX3)) PosY3(length(PosY3));PosX3(length(PosX3)) PosY3(length(PosY3))];
else
    waypoint1=[PosX1(length(PosX1)) PosY1(length(PosY1));PosX1(length(PosX1)) PosY1(length(PosY1))];
    waypoint2=[PosX2(length(PosX2)) PosY2(length(PosY2));PosX2(length(PosX2)) PosY2(length(PosY2))];
    waypoint3=[PosX3(length(PosX3)) PosY3(length(PosY3));PosX3(length(PosX3)) PosY3(length(PosY3))];
end

== matlab function Mtest6/Robot 1/ Extract Goal ==
  data: Waypoints input; Goal output
function Goal = extractGoal(Waypoints)
%#codegen
b = isnan(Waypoints);
[rows,~] = find(b);
ridx = setdiff(1:size(Waypoints,1), sort(rows));
Goal = [Waypoints(ridx(end), 1) Waypoints(ridx(end), 2)];

== matlab function Mtest6/Robot 3/Avoid Collision/Stop Robot On Sensing Obstacles ==
  data: AngleMin input; AngleMax input; angIncrement input; Ranges input; noStop output size=1; avoidCollisionDistance input
function noStop= stopRobot(AngleMin, AngleMax, angIncrement, Ranges, avoidCollisionDistance)
%%stopRobot stops the robot based on the range sensor. 
%   The robot has an on-board range sensor which it uses to detect
%   obstacles. Based: simulateWarehouseRobotInGazebo

%limits on the angle of range readings for defining viewing scope of the robot 
angMin = -pi/10;
angMax = pi/10;

%signal the robot to continue moving unless it sees an obstacle
noStop = true;

%double
range=double(Ranges);
angleMin=double(AngleMin);
angleMax=double(AngleMax);
angleStep=double(angIncrement);
% rawAngles=angleMin:angleStep:angleMax;
numReadings = numel(range);
rawAngles = angleMin + (0:numReadings-1)' * angleStep;
% Wrap the angles to the (-pi,pi] interval.
Angles=robotics.internal.wrapToPi(double(rawAngles));

%if the ray count is non-zero
if true%count ~= 0
    %create a lidar scan object from the range readings
    scan = lidarScan(range, Angles);
    
    %filter out non-zero ranges which are in robot's scope. Range-values are zero if
    %there are no obstacles. 
    % Remove invalid points for refScan (inf/nan + out of range limits)
    rangeScope = removeInvalidData(scan, 'AngleLimits', [angMin angMax]);

%     rangeScope = scan.Ranges((scan.Angles > angMin) & ... 
%                             (scan.Angles < angMax) & ...
%                             (scan.Ranges ~= 0));
                        
    %signal the robot to continue to move if none of the ranges are less than 2m
    noStop = ~any(rangeScope.Ranges < avoidCollisionDistance);
end

end
